simulink model "ackerman_modelo_parte1_neuronal"  (R2023b)
settings: Solver=FixedStepDiscrete  StartTime=0.0  StopTime=50  FixedStep=0.1  RelTol=1e-3
undefined symbols (not defined in the file or in its folder): Angular, Linear
libraries: neural x121, robotlib x15, fuzblock x1, robotcorelib x1
(part 5 of 5)

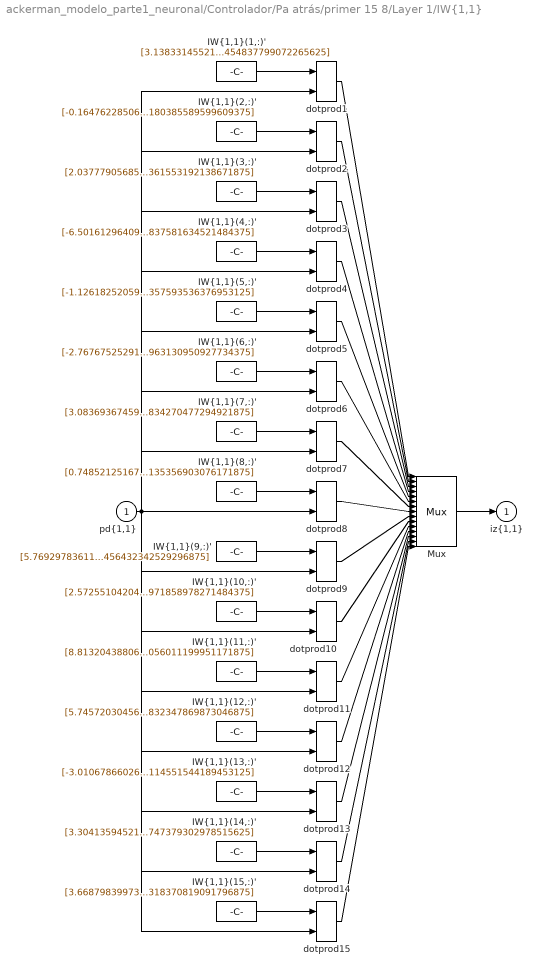
== system ackerman_modelo_parte1_neuronal/Controlador/Pa atrás/primer 15 8/Layer 1/IW{1,1} ==
  "pd{1,1}" : Inport  PortDimensions=12  SampleTime=0.1
      mask Display: e = 0.06;c1 = [120 230 180]/255;c2 = ([120 230 180]+0)/(256+128);c3 = ([120 230 180]+128)/(256+128);patch([0 1 1 0],[0 0 1 1],c1);patch([0 1 1 1-e 1-e 0+e],[0 0 1 1-e 0+e 0+e],c2);patch([0 0 1 1-e 0+e 0+e],[0 1 1 1-e 1-e 0+e],c3);plot([0 1 1 0 0],[0 0 1 1 0]);
  "IW{1,1}(1,:)'" : Constant  Value=[3.13833145521684198087086770101450383663177490234375;-6.19499437988781220809642036329023540019989013671875;-2.00220395313596899455887978547252714633941650390625;-4.82784976961187251021101474179886281490325927734375;5.58430706351398686848597208154387772083282470703125;5.3963459231659864911989643587730824947357177734375;0.0542977229144951945016828176449052989482879638671875;-4.8964896730979479144707511295564472675323486328125;1.547154767949700637785781509592197835445404052734375;7.9004335446761420058692237944342195987701416015625;4.14971538332680278671205087448470294475555419921875;-0.79014433640509429412901454270468093454837799072265625]
      mask Display: e = 0.06;c1 = [120 150 230]/255;c2 = ([120 150 230]+0)/383;c3 = ([120 150 230]+128)/383;patch([0 1 1 0],[0 0 1 1],c1);patch([0 1 1 1-e 1-e 0+e],[0 0 1 1-e 0+e 0+e],c2);patch([0 0 1 1-e 0+e 0+e],[0 1 1 1-e 1-e 0+e],c3);plot([0 1 1 0 0],[0 0 1 1 0]);disp('Weights');
  "IW{1,1}(10,:)'" : Constant  Value=[2.572551042042926727759777350001968443393707275390625;-0.59551225184145584190531508284038864076137542724609375;-0.30685873733525692585999422590248286724090576171875;-2.6996858864094601671013151644729077816009521484375;-4.249827912405418572916460107080638408660888671875;-1.1549695122995402574161971642752178013324737548828125;-13.3261726054552465114966253167949616909027099609375;4.43615378343977084796279086731374263763427734375;0.5770168591797031343304524853010661900043487548828125;0.27150941942864859068862415369949303567409515380859375;3.406433890218272697580914609716273844242095947265625;0.92716581704404477104475290616392157971858978271484375]
      mask Display: e = 0.06;c1 = [120 150 230]/255;c2 = ([120 150 230]+0)/383;c3 = ([120 150 230]+128)/383;patch([0 1 1 0],[0 0 1 1],c1);patch([0 1 1 1-e 1-e 0+e],[0 0 1 1-e 0+e 0+e],c2);patch([0 0 1 1-e 0+e 0+e],[0 1 1 1-e 1-e 0+e],c3);plot([0 1 1 0 0],[0 0 1 1 0]);disp('Weights');
  "IW{1,1}(11,:)'" : Constant  Value=[8.813204388067607197854158584959805011749267578125;-11.7057265338999574311174001195468008518218994140625;-1.1611569417966640660466737244860269129276275634765625;-0.282140073577483274647192956763319671154022216796875;-6.070085924028401080931871547363698482513427734375;-1.1869447949154434684970738089759834110736846923828125;12.797002497650527885753035661764442920684814453125;-6.5006412352421936162727433838881552219390869140625;2.544454447903282900966814850107766687870025634765625;2.772478853294586986777403581072576344013214111328125;3.09454714741394543153774066013284027576446533203125;7.86219239038993134016664043883793056011199951171875]
      mask Display: e = 0.06;c1 = [120 150 230]/255;c2 = ([120 150 230]+0)/383;c3 = ([120 150 230]+128)/383;patch([0 1 1 0],[0 0 1 1],c1);patch([0 1 1 1-e 1-e 0+e],[0 0 1 1-e 0+e 0+e],c2);patch([0 0 1 1-e 0+e 0+e],[0 1 1 1-e 1-e 0+e],c3);plot([0 1 1 0 0],[0 0 1 1 0]);disp('Weights');
  "IW{1,1}(12,:)'" : Constant  Value=[5.7457203045610523162167737609706819057464599609375;-4.95127673804246715150156887830235064029693603515625;-2.57218520303488151768078751047141849994659423828125;-0.73249175551907896863923497221549041569232940673828125;1.6111606945435188453785713136312551796436309814453125;1.1705981175054331888674141737283207476139068603515625;-7.34947786476711684144902392290532588958740234375;-1.7738172654386639148782478514476679265499114990234375;0.5768042451301245154837715745088644325733184814453125;0.224641956192956959714734921362833119928836822509765625;0.3930249748530252329459244720055721700191497802734375;-1.5133229059635364688318759363028220832347869873046875]
      mask Display: e = 0.06;c1 = [120 150 230]/255;c2 = ([120 150 230]+0)/383;c3 = ([120 150 230]+128)/383;patch([0 1 1 0],[0 0 1 1],c1);patch([0 1 1 1-e 1-e 0+e],[0 0 1 1-e 0+e 0+e],c2);patch([0 0 1 1-e 0+e 0+e],[0 1 1 1-e 1-e 0+e],c3);plot([0 1 1 0 0],[0 0 1 1 0]);disp('Weights');
  "IW{1,1}(13,:)'" : Constant  Value=[-3.010678660268370609998100917437113821506500244140625;4.4328891620700812126187884132377803325653076171875;5.807431661847648030061463941819965839385986328125;3.476791359428748950932686057058162987232208251953125;2.4697341429991155337120289914309978485107421875;2.05477310015384961872086932999081909656524658203125;-1.5218585447957073686353623998002149164676666259765625;1.324210651061530352734507687273435294628143310546875;5.75386815156350195366030675359070301055908203125;5.10401477499944977722634575911797583103179931640625;1.7878470401743256079640786992968060076236724853515625;-1.4389725445316703389408985458430834114551544189453125]
      mask Display: e = 0.06;c1 = [120 150 230]/255;c2 = ([120 150 230]+0)/383;c3 = ([120 150 230]+128)/383;patch([0 1 1 0],[0 0 1 1],c1);patch([0 1 1 1-e 1-e 0+e],[0 0 1 1-e 0+e 0+e],c2);patch([0 0 1 1-e 0+e 0+e],[0 1 1 1-e 1-e 0+e],c3);plot([0 1 1 0 0],[0 0 1 1 0]);disp('Weights');
  "IW{1,1}(14,:)'" : Constant  Value=[3.3041359452168297394791807164438068866729736328125;0.1762778979927372702274368521102587692439556121826171875;5.4050963927401287634211257682181894779205322265625;-3.18648301109764275906854891218245029449462890625;0.5385228763760065984200764432898722589015960693359375;-2.302199268748124527661502725095488131046295166015625;5.49227092147563933366427590954117476940155029296875;0.97919070401553154336937723201117478311061859130859375;1.145084516988541967208448113524354994297027587890625;4.27032650445300010488836051081307232379913330078125;1.6231956725708138744579400736256502568721771240234375;-0.6865005967335078285174176926375366747379302978515625]
      mask Display: e = 0.06;c1 = [120 150 230]/255;c2 = ([120 150 230]+0)/383;c3 = ([120 150 230]+128)/383;patch([0 1 1 0],[0 0 1 1],c1);patch([0 1 1 1-e 1-e 0+e],[0 0 1 1-e 0+e 0+e],c2);patch([0 0 1 1-e 0+e 0+e],[0 1 1 1-e 1-e 0+e],c3);plot([0 1 1 0 0],[0 0 1 1 0]);disp('Weights');
  "IW{1,1}(15,:)'" : Constant  Value=[3.668798399734122472892750010942108929157257080078125;-5.38938465059415960922706290148198604583740234375;-3.401566331543757204514122349792160093784332275390625;-1.1609126490613366211590573584544472396373748779296875;6.618010649271667489301762543618679046630859375;-7.862741094876252390122317592613399028778076171875;3.54191550708989755236189012066461145877838134765625;-1.3477909930119469361642359217512421309947967529296875;1.9546134173191365146493581050890497863292694091796875;-1.1566749706934935648661166851525194942951202392578125;2.921489032247831740818355683586560189723968505859375;1.5151945125394365998516832405584864318370819091796875]
      mask Display: e = 0.06;c1 = [120 150 230]/255;c2 = ([120 150 230]+0)/383;c3 = ([120 150 230]+128)/383;patch([0 1 1 0],[0 0 1 1],c1);patch([0 1 1 1-e 1-e 0+e],[0 0 1 1-e 0+e 0+e],c2);patch([0 0 1 1-e 0+e 0+e],[0 1 1 1-e 1-e 0+e],c3);plot([0 1 1 0 0],[0 0 1 1 0]);disp('Weights');
  "IW{1,1}(2,:)'" : Constant  Value=[-0.1647622850618779555276205428526736795902252197265625;-6.67270935708041523781730575137771666049957275390625;-1.6748440892445206618077691018697805702686309814453125;0.97276097993890042747722191052162088453769683837890625;2.73413105911384235469085979275405406951904296875;-4.61712661552317182867000155965797603130340576171875;-2.911426019223313677031228507985360920429229736328125;0.72363976938584340103943759459070861339569091796875;-0.98313354310142819780793388417805545032024383544921875;-2.691014741691610812068802260910160839557647705078125;4.420274579392863500970634049735963344573974609375;-3.880848224433525839316416750079952180385589599609375]
      mask Display: e = 0.06;c1 = [120 150 230]/255;c2 = ([120 150 230]+0)/383;c3 = ([120 150 230]+128)/383;patch([0 1 1 0],[0 0 1 1],c1);patch([0 1 1 1-e 1-e 0+e],[0 0 1 1-e 0+e 0+e],c2);patch([0 0 1 1-e 0+e 0+e],[0 1 1 1-e 1-e 0+e],c3);plot([0 1 1 0 0],[0 0 1 1 0]);disp('Weights');
  "IW{1,1}(3,:)'" : Constant  Value=[2.03777905685296989446442239568568766117095947265625;-2.160035947260035005257350348983891308307647705078125;2.605648632233163564109190701856277883052825927734375;2.3092568544783862449776279390789568424224853515625;3.3144277547602793987380209728144109249114990234375;-2.28108752553862448309018873260356485843658447265625;-10.7986674070768398081554551026783883571624755859375;3.853720755030112687933296911069191992282867431640625;-2.361428195660809858935635929810814559459686279296875;-3.596462160164643595550160171114839613437652587890625;-3.910945166775002146408724001958034932613372802734375;-2.429732741520268302082286027143709361553192138671875]
      mask Display: e = 0.06;c1 = [120 150 230]/255;c2 = ([120 150 230]+0)/383;c3 = ([120 150 230]+128)/383;patch([0 1 1 0],[0 0 1 1],c1);patch([0 1 1 1-e 1-e 0+e],[0 0 1 1-e 0+e 0+e],c2);patch([0 0 1 1-e 0+e 0+e],[0 1 1 1-e 1-e 0+e],c3);plot([0 1 1 0 0],[0 0 1 1 0]);disp('Weights');
  "IW{1,1}(4,:)'" : Constant  Value=[-6.5016129640967559311093282303772866725921630859375;-0.79522721813868890716747728220070712268352508544921875;-6.73803458296746260458576216478832066059112548828125;-3.476541997292326602320144957047887146472930908203125;-2.55914140829384084696584977791644632816314697265625;-3.88475771154622950831480920896865427494049072265625;-1.4635945598190376326641626292257569730281829833984375;3.299453679629163360687016393058001995086669921875;3.0582672371355261731196151231415569782257080078125;-0.57414285366964612489226738034631125628948211669921875;0.93060935916938891665495248162187635898590087890625;-0.429906101754307046203251729821204207837581634521484375]
      mask Display: e = 0.06;c1 = [120 150 230]/255;c2 = ([120 150 230]+0)/383;c3 = ([120 150 230]+128)/383;patch([0 1 1 0],[0 0 1 1],c1);patch([0 1 1 1-e 1-e 0+e],[0 0 1 1-e 0+e 0+e],c2);patch([0 0 1 1-e 0+e 0+e],[0 1 1 1-e 1-e 0+e],c3);plot([0 1 1 0 0],[0 0 1 1 0]);disp('Weights');
  "IW{1,1}(5,:)'" : Constant  Value=[-1.126182520599181113851727786823175847530364990234375;-0.67009231564694093918888029293157160282135009765625;2.990487179943574158613728286582045257091522216796875;1.686459004262194749657055581337772309780120849609375;-0.51295798280588311701677639575791545212268829345703125;-0.1693192751783541283305822844340582378208637237548828125;-3.36835087006842837098474774393253028392791748046875;3.730050960124993597588627380901016294956207275390625;1.9196643529733361521749657185864634811878204345703125;1.694496082969093375680813551298342645168304443359375;-1.0729297441333509599559192793094553053379058837890625;-2.796374710798151586033100102213211357593536376953125]
      mask Display: e = 0.06;c1 = [120 150 230]/255;c2 = ([120 150 230]+0)/383;c3 = ([120 150 230]+128)/383;patch([0 1 1 0],[0 0 1 1],c1);patch([0 1 1 1-e 1-e 0+e],[0 0 1 1-e 0+e 0+e],c2);patch([0 0 1 1-e 0+e 0+e],[0 1 1 1-e 1-e 0+e],c3);plot([0 1 1 0 0],[0 0 1 1 0]);disp('Weights');
  "IW{1,1}(6,:)'" : Constant  Value=[-2.767675252918380568445400058408267796039581298828125;-7.073354838042828163224839954636991024017333984375;-1.3531578339525538456911135654081590473651885986328125;-3.06300573535806019975780145614407956600189208984375;-7.13075550648704403755573366652242839336395263671875;-3.744633843247024973521774882101453840732574462890625;-8.208592620912252613152304547838866710662841796875;2.46583543118132553217947133816778659820556640625;-3.340073357912283658066598945879377424716949462890625;-2.799475440893957500776423330535180866718292236328125;-2.249013441580913319484125167946331202983856201171875;2.392302749944286599514953195466659963130950927734375]
      mask Display: e = 0.06;c1 = [120 150 230]/255;c2 = ([120 150 230]+0)/383;c3 = ([120 150 230]+128)/383;patch([0 1 1 0],[0 0 1 1],c1);patch([0 1 1 1-e 1-e 0+e],[0 0 1 1-e 0+e 0+e],c2);patch([0 0 1 1-e 0+e 0+e],[0 1 1 1-e 1-e 0+e],c3);plot([0 1 1 0 0],[0 0 1 1 0]);disp('Weights');
  "IW{1,1}(7,:)'" : Constant  Value=[3.0836936745987717500838698470033705234527587890625;-0.88318704317611373966201426810584962368011474609375;1.7110761895791217757079039074596948921680450439453125;-0.31400445778907759564191337631200440227985382080078125;2.64346625227536247138004910084418952465057373046875;-0.6176657494047643748302789390436373651027679443359375;-0.63152317856311934729518497988465242087841033935546875;8.3510900927338820309842049027793109416961669921875;-5.97435811941152916659802940557710826396942138671875;-0.6339005945491880122943939568358473479747772216796875;2.279868767326854506194422356202267110347747802734375;-3.37930106039398037154342091525904834270477294921875]
      mask Display: e = 0.06;c1 = [120 150 230]/255;c2 = ([120 150 230]+0)/383;c3 = ([120 150 230]+128)/383;patch([0 1 1 0],[0 0 1 1],c1);patch([0 1 1 1-e 1-e 0+e],[0 0 1 1-e 0+e 0+e],c2);patch([0 0 1 1-e 0+e 0+e],[0 1 1 1-e 1-e 0+e],c3);plot([0 1 1 0 0],[0 0 1 1 0]);disp('Weights');
  "IW{1,1}(8,:)'" : Constant  Value=[0.74852125167156613461116876351297833025455474853515625;-4.012567271762879528296252829022705554962158203125;1.0633341155585138704253722607973031699657440185546875;-0.58494336521590450939100946925464086234569549560546875;-0.5453224736011679230074378210701979696750640869140625;3.469959956693179581321828663931228220462799072265625;-5.89367912672649563177174059092067182064056396484375;-4.74017192421732413976087627816013991832733154296875;-4.9750537290780183496963218203745782375335693359375;6.49748859653846633221974116167984902858734130859375;-1.910694940986072065669532094034366309642791748046875;-2.236924241129784274306757652084343135356903076171875]
      mask Display: e = 0.06;c1 = [120 150 230]/255;c2 = ([120 150 230]+0)/383;c3 = ([120 150 230]+128)/383;patch([0 1 1 0],[0 0 1 1],c1);patch([0 1 1 1-e 1-e 0+e],[0 0 1 1-e 0+e 0+e],c2);patch([0 0 1 1-e 0+e 0+e],[0 1 1 1-e 1-e 0+e],c3);plot([0 1 1 0 0],[0 0 1 1 0]);disp('Weights');
  "IW{1,1}(9,:)'" : Constant  Value=[5.76929783611728819181507788016460835933685302734375;0.85907947622363323159078163371304981410503387451171875;-1.0414871446960243250856592567288316786289215087890625;-0.60378548209747384678536263891146518290042877197265625;1.936814065109272231524073504260741174221038818359375;5.14869148164522183463986948481760919094085693359375;-1.94708708587885492846680790535174310207366943359375;-0.52074196027196240077472566554206423461437225341796875;1.6221727344143810345400424921535886824131011962890625;-1.153231367094303738696225991589017212390899658203125;0.47589760448268070280875008393195457756519317626953125;1.595810956015813797392866035806946456432342529296875]
      mask Display: e = 0.06;c1 = [120 150 230]/255;c2 = ([120 150 230]+0)/383;c3 = ([120 150 230]+128)/383;patch([0 1 1 0],[0 0 1 1],c1);patch([0 1 1 1-e 1-e 0+e],[0 0 1 1-e 0+e 0+e],c2);patch([0 0 1 1-e 0+e 0+e],[0 1 1 1-e 1-e 0+e],c3);plot([0 1 1 0 0],[0 0 1 1 0]);disp('Weights');
  Mux : Mux  Inputs=15
      mask Display: e = 0.06;c1 = [120 150 230]/255;c2 = ([120 150 230]+0)/383;c3 = ([120 150 230]+128)/383;patch([0 1 1 0],[0 0 1 1],c1);patch([0 1 1 1-e 1-e 0+e],[0 0 1 1-e 0+e 0+e],c2);patch([0 0 1 1-e 0+e 0+e],[0 1 1 1-e 1-e 0+e],c3);plot([0 1 1 0 0],[0 0 1 1 0]);disp('Mux');
  dotprod{1..15} (15 alike) : neural/Weight Functions/dotprod
  "iz{1,1}" : Outport
      mask Display: e = 0.06;c1 = [120 230 180]/255;c2 = ([120 230 180]+0)/(256+128);c3 = ([120 230 180]+128)/(256+128);patch([0 1 1 0],[0 0 1 1],c1);patch([0 1 1 1-e 1-e 0+e],[0 0 1 1-e 0+e 0+e],c2);patch([0 0 1 1-e 0+e 0+e],[0 1 1 1-e 1-e 0+e],c3);plot([0 1 1 0 0],[0 0 1 1 0]);
  wires:
  Mux/1 -> "iz{1,1}"/1
  dotprod15/1 -> Mux/15
  "IW{1,1}(15,:)'"/1 -> dotprod15/1
  dotprod14/1 -> Mux/14
  "IW{1,1}(14,:)'"/1 -> dotprod14/1
  dotprod13/1 -> Mux/13
  "IW{1,1}(13,:)'"/1 -> dotprod13/1
  dotprod12/1 -> Mux/12
  "IW{1,1}(12,:)'"/1 -> dotprod12/1
  dotprod11/1 -> Mux/11
  "IW{1,1}(11,:)'"/1 -> dotprod11/1
  dotprod10/1 -> Mux/10
  "IW{1,1}(10,:)'"/1 -> dotprod10/1
  dotprod9/1 -> Mux/9
  "IW{1,1}(9,:)'"/1 -> dotprod9/1
  dotprod8/1 -> Mux/8
  "IW{1,1}(8,:)'"/1 -> dotprod8/1
  dotprod7/1 -> Mux/7
  "IW{1,1}(7,:)'"/1 -> dotprod7/1
  dotprod6/1 -> Mux/6
  "IW{1,1}(6,:)'"/1 -> dotprod6/1
  dotprod5/1 -> Mux/5
  "IW{1,1}(5,:)'"/1 -> dotprod5/1
  dotprod4/1 -> Mux/4
  "IW{1,1}(4,:)'"/1 -> dotprod4/1
  dotprod3/1 -> Mux/3
  "IW{1,1}(3,:)'"/1 -> dotprod3/1
  dotprod2/1 -> Mux/2
  "IW{1,1}(2,:)'"/1 -> dotprod2/1
  dotprod1/1 -> Mux/1
  "pd{1,1}"/1 -> dotprod15/2, dotprod14/2, dotprod13/2, dotprod12/2, dotprod11/2, dotprod10/2, dotprod9/2, dotprod8/2, dotprod7/2, dotprod6/2, dotprod5/2, dotprod4/2, dotprod3/2, dotprod2/2, dotprod1/2
  "IW{1,1}(1,:)'"/1 -> dotprod1/1

== system ackerman_modelo_parte1_neuronal/Controlador/Pa atrás/primer 15 8/Layer 2/Delays 1 ==
  "p{2}" : Inport  PortDimensions=15  SampleTime=0.1
      mask Display: e = 0.06;c1 = [120 230 180]/255;c2 = ([120 230 180]+0)/(256+128);c3 = ([120 230 180]+128)/(256+128);patch([0 1 1 0],[0 0 1 1],c1);patch([0 1 1 1-e 1-e 0+e],[0 0 1 1-e 0+e 0+e],c2);patch([0 0 1 1-e 0+e 0+e],[0 1 1 1-e 1-e 0+e],c3);plot([0 1 1 0 0],[0 0 1 1 0]);
  mux : Mux  Inputs=1
      mask Display: e = 0.06;c1 = [120 150 230]/255;c2 = ([120 150 230]+0)/383;c3 = ([120 150 230]+128)/383;patch([0 1 1 0],[0 0 1 1],c1);patch([0 1 1 1-e 1-e 0+e],[0 0 1 1-e 0+e 0+e],c2);patch([0 0 1 1-e 0+e 0+e],[0 1 1 1-e 1-e 0+e],c3);plot([0 1 1 0 0],[0 0 1 1 0]);disp('Mux')
  "pd{2,1}" : Outport
      mask Display: e = 0.06;c1 = [120 230 180]/255;c2 = ([120 230 180]+0)/(256+128);c3 = ([120 230 180]+128)/(256+128);patch([0 1 1 0],[0 0 1 1],c1);patch([0 1 1 1-e 1-e 0+e],[0 0 1 1-e 0+e 0+e],c2);patch([0 0 1 1-e 0+e 0+e],[0 1 1 1-e 1-e 0+e],c3);plot([0 1 1 0 0],[0 0 1 1 0]);
  wires:
  mux/1 -> "pd{2,1}"/1
  "p{2}"/1 -> mux/1

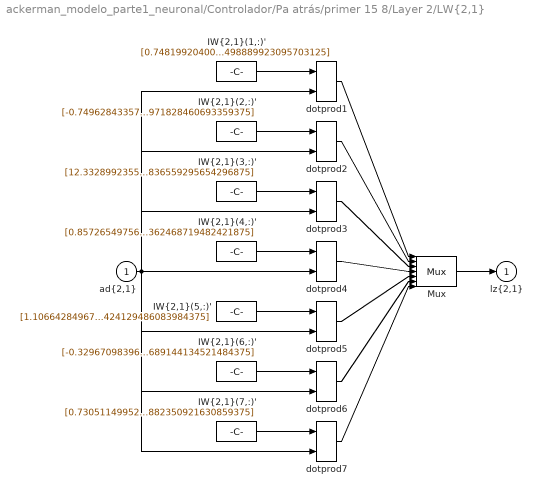
== system ackerman_modelo_parte1_neuronal/Controlador/Pa atrás/primer 15 8/Layer 2/LW{2,1} ==
  "ad{2,1}" : Inport  PortDimensions=15  SampleTime=0.1
      mask Display: e = 0.06;c1 = [120 230 180]/255;c2 = ([120 230 180]+0)/(256+128);c3 = ([120 230 180]+128)/(256+128);patch([0 1 1 0],[0 0 1 1],c1);patch([0 1 1 1-e 1-e 0+e],[0 0 1 1-e 0+e 0+e],c2);patch([0 0 1 1-e 0+e 0+e],[0 1 1 1-e 1-e 0+e],c3);plot([0 1 1 0 0],[0 0 1 1 0]);
  "IW{2,1}(1,:)'" : Constant  Value=[0.7481992040039153746278088874532841145992279052734375;-1.126597024044754480343044633627869188785552978515625;1.5155775237853175152480389442644082009792327880859375;2.0469156099994307851375197060406208038330078125;7.8138659751533072750362407532520592212677001953125;2.903583859678425138639568103826604783535003662109375;1.6622982814302422749364041010267101228237152099609375;5.9303213640288259256294622900895774364471435546875;-4.31311558360107927256876791943795979022979736328125;-8.8773576403826783831618740805424749851226806640625;-4.04397070113652556955230465973727405071258544921875;-5.08185092549631800551424021250568330287933349609375;-2.80925265953370395521915270364843308925628662109375;-1.864831680495824262067117160768248140811920166015625;2.65513075966677281058991866302676498889923095703125]
      mask Display: e = 0.06;c1 = [120 150 230]/255;c2 = ([120 150 230]+0)/383;c3 = ([120 150 230]+128)/383;patch([0 1 1 0],[0 0 1 1],c1);patch([0 1 1 1-e 1-e 0+e],[0 0 1 1-e 0+e 0+e],c2);patch([0 0 1 1-e 0+e 0+e],[0 1 1 1-e 1-e 0+e],c3);plot([0 1 1 0 0],[0 0 1 1 0]);disp('weights');
  "IW{2,1}(2,:)'" : Constant  Value=[-0.74962843357484931772205527522601187229156494140625;-6.93165936727352960389225700055249035358428955078125;-4.01275508893955379363660540548153221607208251953125;-2.120531649750461600234530123998410999774932861328125;1.829294262234303136693824853864498436450958251953125;6.57831915986466153611900153919123113155364990234375;3.111129228600808982463377105887047946453094482421875;-1.906397126721314894126635408611036837100982666015625;-2.561940433343730116888536940678022801876068115234375;3.701734633273577212975169459241442382335662841796875;2.456765678314351664113246442866511642932891845703125;-0.88958234176935591097645783520420081913471221923828125;-6.4768830231558265353442038758657872676849365234375;4.57889656160470082113533862866461277008056640625;4.0829006341815610170442596427164971828460693359375]
      mask Display: e = 0.06;c1 = [120 150 230]/255;c2 = ([120 150 230]+0)/383;c3 = ([120 150 230]+128)/383;patch([0 1 1 0],[0 0 1 1],c1);patch([0 1 1 1-e 1-e 0+e],[0 0 1 1-e 0+e 0+e],c2);patch([0 0 1 1-e 0+e 0+e],[0 1 1 1-e 1-e 0+e],c3);plot([0 1 1 0 0],[0 0 1 1 0]);disp('weights');
  "IW{2,1}(3,:)'" : Constant  Value=[12.3328992355445858919438251177780330181121826171875;11.0004326759787804945744937867857515811920166015625;-5.34841924221345532686200385796837508678436279296875;-7.0994335148749936337253529927693307399749755859375;2.263077368879132134082965421839617192745208740234375;-7.31242298972578996796300998539663851261138916015625;9.365048931524153630334694753400981426239013671875;3.968973565914051704339726711623370647430419921875;15.059144497544654228704530396498739719390869140625;6.4716573827061711909891528193838894367218017578125;-5.9158271638871067210629917099140584468841552734375;-3.05024650789953444274260618840344250202178955078125;8.2370518811566935113432919024489820003509521484375;-11.6324162769302521525105476030148565769195556640625;2.01322611861408784506011215853504836559295654296875]
      mask Display: e = 0.06;c1 = [120 150 230]/255;c2 = ([120 150 230]+0)/383;c3 = ([120 150 230]+128)/383;patch([0 1 1 0],[0 0 1 1],c1);patch([0 1 1 1-e 1-e 0+e],[0 0 1 1-e 0+e 0+e],c2);patch([0 0 1 1-e 0+e 0+e],[0 1 1 1-e 1-e 0+e],c3);plot([0 1 1 0 0],[0 0 1 1 0]);disp('weights');
  "IW{2,1}(4,:)'" : Constant  Value=[0.85726549756485825870555572691955603659152984619140625;-1.6157874357042329993561224910081364214420318603515625;-2.3378881600398013773656202829442918300628662109375;1.4068312031528831251847577732405625283718109130859375;1.1609880290264327218352491399855352938175201416015625;5.043137081505467023134769988246262073516845703125;1.6282908256337644825606503218295983970165252685546875;0.9851818610864018221917604023474268615245819091796875;-1.5742354980467549996347997876000590622425079345703125;-6.4182878725017058485491361352615058422088623046875;1.236131349069788054606533478363417088985443115234375;-1.5151875690311220612471743152127601206302642822265625;-5.4046776681074533144055749289691448211669921875;-0.301835111587298310364957387719186954200267791748046875;-1.662398546290766443433994936640374362468719482421875]
      mask Display: e = 0.06;c1 = [120 150 230]/255;c2 = ([120 150 230]+0)/383;c3 = ([120 150 230]+128)/383;patch([0 1 1 0],[0 0 1 1],c1);patch([0 1 1 1-e 1-e 0+e],[0 0 1 1-e 0+e 0+e],c2);patch([0 0 1 1-e 0+e 0+e],[0 1 1 1-e 1-e 0+e],c3);plot([0 1 1 0 0],[0 0 1 1 0]);disp('weights');
  "IW{2,1}(5,:)'" : Constant  Value=[1.106642849674602135934264879324473440647125244140625;0.571502015897777937425416894257068634033203125;0.81620295508666396155916800125851295888423919677734375;-3.915085877175725759258284597308374941349029541015625;1.7182548217798458978222697624005377292633056640625;-0.932288532598022801067827458609826862812042236328125;-3.802149167051169786901709812809713184833526611328125;1.1218625349822100023544635405414737761020660400390625;1.2108603063697682689081602802616544067859649658203125;-1.3837647454165533655867648121784441173076629638671875;-2.294782958455342747328131736139766871929168701171875;0.27139709347339202594184826011769473552703857421875;0.35111556880865635310584593753446824848651885986328125;-0.535119520474186316505438298918306827545166015625;0.177795112653033215988074289271025918424129486083984375]
      mask Display: e = 0.06;c1 = [120 150 230]/255;c2 = ([120 150 230]+0)/383;c3 = ([120 150 230]+128)/383;patch([0 1 1 0],[0 0 1 1],c1);patch([0 1 1 1-e 1-e 0+e],[0 0 1 1-e 0+e 0+e],c2);patch([0 0 1 1-e 0+e 0+e],[0 1 1 1-e 1-e 0+e],c3);plot([0 1 1 0 0],[0 0 1 1 0]);disp('weights');
  "IW{2,1}(6,:)'" : Constant  Value=[-0.329670983964105934749255766291753388941287994384765625;0.9447396245833641348355058653396554291248321533203125;-0.260196034449015456413434321802924387156963348388671875;-0.2872857726077722162472127820365130901336669921875;2.91913437532715480671186014660634100437164306640625;0.1852331668108104789638446163735352456569671630859375;0.68985458226234264156317976812715642154216766357421875;-1.7856832233152906130868586842552758753299713134765625;-0.44000187852971850421823774013319052755832672119140625;-2.142873037757759835386650593136437237262725830078125;0.388272349961649665406326903394074179232120513916015625;-0.60718998768551724065645203154417686164379119873046875;0.8371629651469361110827094307751394808292388916015625;0.1650951326068933744384281681050197221338748931884765625;0.64000300449640989963739912127493880689144134521484375]
      mask Display: e = 0.06;c1 = [120 150 230]/255;c2 = ([120 150 230]+0)/383;c3 = ([120 150 230]+128)/383;patch([0 1 1 0],[0 0 1 1],c1);patch([0 1 1 1-e 1-e 0+e],[0 0 1 1-e 0+e 0+e],c2);patch([0 0 1 1-e 0+e 0+e],[0 1 1 1-e 1-e 0+e],c3);plot([0 1 1 0 0],[0 0 1 1 0]);disp('weights');
  "IW{2,1}(7,:)'" : Constant  Value=[0.73051149952431082557069430549745447933673858642578125;3.05826356477004512868234087363816797733306884765625;-1.673669437076252819451838149689137935638427734375;-2.400459004009674490731640617013908922672271728515625;-9.80319466489697077804521541111171245574951171875;4.62435712954842959021561910049058496952056884765625;-4.84177000897603448947847937233746051788330078125;-8.425474797648991653886696440167725086212158203125;-3.37578421790337568353379538166336715221405029296875;-3.11041385548329518684340655454434454441070556640625;2.677786696924715936773964131134562194347381591796875;3.9061912060113375133596491650678217411041259765625;1.013606829036505008190260923583991825580596923828125;4.45431275129676151891544577665627002716064453125;-10.9998218846045059393645715317688882350921630859375]
      mask Display: e = 0.06;c1 = [120 150 230]/255;c2 = ([120 150 230]+0)/383;c3 = ([120 150 230]+128)/383;patch([0 1 1 0],[0 0 1 1],c1);patch([0 1 1 1-e 1-e 0+e],[0 0 1 1-e 0+e 0+e],c2);patch([0 0 1 1-e 0+e 0+e],[0 1 1 1-e 1-e 0+e],c3);plot([0 1 1 0 0],[0 0 1 1 0]);disp('weights');
  Mux : Mux  Inputs=7
      mask Display: e = 0.06;c1 = [120 150 230]/255;c2 = ([120 150 230]+0)/383;c3 = ([120 150 230]+128)/383;patch([0 1 1 0],[0 0 1 1],c1);patch([0 1 1 1-e 1-e 0+e],[0 0 1 1-e 0+e 0+e],c2);patch([0 0 1 1-e 0+e 0+e],[0 1 1 1-e 1-e 0+e],c3);plot([0 1 1 0 0],[0 0 1 1 0]);disp('Mux');
  dotprod{1..7} (7 alike) : neural/Weight Functions/dotprod
  "lz{2,1}" : Outport
      mask Display: e = 0.06;c1 = [120 230 180]/255;c2 = ([120 230 180]+0)/(256+128);c3 = ([120 230 180]+128)/(256+128);patch([0 1 1 0],[0 0 1 1],c1);patch([0 1 1 1-e 1-e 0+e],[0 0 1 1-e 0+e 0+e],c2);patch([0 0 1 1-e 0+e 0+e],[0 1 1 1-e 1-e 0+e],c3);plot([0 1 1 0 0],[0 0 1 1 0]);
  wires:
  Mux/1 -> "lz{2,1}"/1
  dotprod7/1 -> Mux/7
  "IW{2,1}(7,:)'"/1 -> dotprod7/1
  dotprod6/1 -> Mux/6
  "IW{2,1}(6,:)'"/1 -> dotprod6/1
  dotprod5/1 -> Mux/5
  "IW{2,1}(5,:)'"/1 -> dotprod5/1
  dotprod4/1 -> Mux/4
  "IW{2,1}(4,:)'"/1 -> dotprod4/1
  dotprod3/1 -> Mux/3
  "IW{2,1}(3,:)'"/1 -> dotprod3/1
  dotprod2/1 -> Mux/2
  "IW{2,1}(2,:)'"/1 -> dotprod2/1
  dotprod1/1 -> Mux/1
  "ad{2,1}"/1 -> dotprod7/2, dotprod6/2, dotprod5/2, dotprod4/2, dotprod3/2, dotprod2/2, dotprod1/2
  "IW{2,1}(1,:)'"/1 -> dotprod1/1

== system ackerman_modelo_parte1_neuronal/Controlador/Pa atrás/primer 15 8/Layer 3/Delays 1 ==
  "p{3}" : Inport  PortDimensions=7  SampleTime=0.1
      mask Display: e = 0.06;c1 = [120 230 180]/255;c2 = ([120 230 180]+0)/(256+128);c3 = ([120 230 180]+128)/(256+128);patch([0 1 1 0],[0 0 1 1],c1);patch([0 1 1 1-e 1-e 0+e],[0 0 1 1-e 0+e 0+e],c2);patch([0 0 1 1-e 0+e 0+e],[0 1 1 1-e 1-e 0+e],c3);plot([0 1 1 0 0],[0 0 1 1 0]);
  mux : Mux  Inputs=1
      mask Display: e = 0.06;c1 = [120 150 230]/255;c2 = ([120 150 230]+0)/383;c3 = ([120 150 230]+128)/383;patch([0 1 1 0],[0 0 1 1],c1);patch([0 1 1 1-e 1-e 0+e],[0 0 1 1-e 0+e 0+e],c2);patch([0 0 1 1-e 0+e 0+e],[0 1 1 1-e 1-e 0+e],c3);plot([0 1 1 0 0],[0 0 1 1 0]);disp('Mux')
  "pd{3,2}" : Outport
      mask Display: e = 0.06;c1 = [120 230 180]/255;c2 = ([120 230 180]+0)/(256+128);c3 = ([120 230 180]+128)/(256+128);patch([0 1 1 0],[0 0 1 1],c1);patch([0 1 1 1-e 1-e 0+e],[0 0 1 1-e 0+e 0+e],c2);patch([0 0 1 1-e 0+e 0+e],[0 1 1 1-e 1-e 0+e],c3);plot([0 1 1 0 0],[0 0 1 1 0]);
  wires:
  mux/1 -> "pd{3,2}"/1
  "p{3}"/1 -> mux/1

== system ackerman_modelo_parte1_neuronal/Controlador/Pa atrás/primer 15 8/Layer 3/LW{3,2} ==
  "ad{3,2}" : Inport  PortDimensions=7  SampleTime=0.1
      mask Display: e = 0.06;c1 = [120 230 180]/255;c2 = ([120 230 180]+0)/(256+128);c3 = ([120 230 180]+128)/(256+128);patch([0 1 1 0],[0 0 1 1],c1);patch([0 1 1 1-e 1-e 0+e],[0 0 1 1-e 0+e 0+e],c2);patch([0 0 1 1-e 0+e 0+e],[0 1 1 1-e 1-e 0+e],c3);plot([0 1 1 0 0],[0 0 1 1 0]);
  "IW{3,2}(1,:)'" : Constant  Value=[-0.264079440465544046379164910831605084240436553955078125;0.51230046191857103732303357901400886476039886474609375;-0.6652775182707999501730000702082179486751556396484375;-0.53484339021644611289474369186791591346263885498046875;-0.149228947666670774818697964292368851602077484130859375;-0.008433135735000978072672950247579137794673442840576171875;-0.85256293215924350281653687488869763910770416259765625]
      mask Display: e = 0.06;c1 = [120 150 230]/255;c2 = ([120 150 230]+0)/383;c3 = ([120 150 230]+128)/383;patch([0 1 1 0],[0 0 1 1],c1);patch([0 1 1 1-e 1-e 0+e],[0 0 1 1-e 0+e 0+e],c2);patch([0 0 1 1-e 0+e 0+e],[0 1 1 1-e 1-e 0+e],c3);plot([0 1 1 0 0],[0 0 1 1 0]);disp('weights');
  "IW{3,2}(2,:)'" : Constant  Value=[0.445211164821717797490663315329584293067455291748046875;0.2497172286753712444618003019058960489928722381591796875;0.24675394014089579997062173788435757160186767578125;-0.017453169559885635397922243328139302320778369903564453125;-0.534125695750038431697248597629368305206298828125;0.041939997232147328831697308260118006728589534759521484375;0.475153394142820373335922568003297783434391021728515625]
      mask Display: e = 0.06;c1 = [120 150 230]/255;c2 = ([120 150 230]+0)/383;c3 = ([120 150 230]+128)/383;patch([0 1 1 0],[0 0 1 1],c1);patch([0 1 1 1-e 1-e 0+e],[0 0 1 1-e 0+e 0+e],c2);patch([0 0 1 1-e 0+e 0+e],[0 1 1 1-e 1-e 0+e],c3);plot([0 1 1 0 0],[0 0 1 1 0]);disp('weights');
  Mux : Mux  Inputs=2
      mask Display: e = 0.06;c1 = [120 150 230]/255;c2 = ([120 150 230]+0)/383;c3 = ([120 150 230]+128)/383;patch([0 1 1 0],[0 0 1 1],c1);patch([0 1 1 1-e 1-e 0+e],[0 0 1 1-e 0+e 0+e],c2);patch([0 0 1 1-e 0+e 0+e],[0 1 1 1-e 1-e 0+e],c3);plot([0 1 1 0 0],[0 0 1 1 0]);disp('Mux');
  dotprod1 : neural/Weight Functions/dotprod
  dotprod2 : neural/Weight Functions/dotprod
  "lz{3,2}" : Outport
      mask Display: e = 0.06;c1 = [120 230 180]/255;c2 = ([120 230 180]+0)/(256+128);c3 = ([120 230 180]+128)/(256+128);patch([0 1 1 0],[0 0 1 1],c1);patch([0 1 1 1-e 1-e 0+e],[0 0 1 1-e 0+e 0+e],c2);patch([0 0 1 1-e 0+e 0+e],[0 1 1 1-e 1-e 0+e],c3);plot([0 1 1 0 0],[0 0 1 1 0]);
  wires:
  Mux/1 -> "lz{3,2}"/1
  dotprod2/1 -> Mux/2
  "IW{3,2}(2,:)'"/1 -> dotprod2/1
  dotprod1/1 -> Mux/1
  "ad{3,2}"/1 -> dotprod2/2, dotprod1/2
  "IW{3,2}(1,:)'"/1 -> dotprod1/1

== matlab function ackerman_modelo_parte1_neuronal/ROS Robot/Conversion_diff_ackerman ==
  data: steering_wheel_angle input; V output; linear_vel_ackerman_kmh input; W output
function [V,W] = fcn(steering_wheel_angle, linear_vel_ackerman_kmh)

    %Aproximacion de angulo volante y velocidad linal a vel_linar y angular.
    % *************************************
    
    min_turning_radius_vehicle = 2;  % radio de giro del vehiculo. Radio minimo en el que gira 180 grados. 
    max_turning_radius_vehicle = 34; % radio de giro del vehiculo. Radio máximo con el volante girado 1º
    max_steering_wheel_angle = 90;  % angulo máximo de volante permitido (grados).
    max_vehicle_linear_speed = 30;  % velocidad máxima de vehiculo (km/h).
    
    
    % Filtrado des los valores máximos
    
    if steering_wheel_angle > max_steering_wheel_angle
        steering_wheel_angle = max_steering_wheel_angle;  
    end
    
    if steering_wheel_angle < (-1*max_steering_wheel_angle)
        steering_wheel_angle = max_steering_wheel_angle;  
    end
    
    if linear_vel_ackerman_kmh > max_vehicle_linear_speed
        linear_vel_ackerman_kmh = max_vehicle_linear_speed;
    end
    
    
    %Conversion a m/s
    linear_vel_ackerman_ms = linear_vel_ackerman_kmh/3.6; %(m/s)
    
    %Conversion a linear and angular velocity for the simulator.
    % v=rω --> ω = v/r
    
    % max_steering_wheel_angle -- > min_turning_radius_vehicle
    % steering_wheel_angle = 0 --> angular_vel_vehicle = 0;
    
    turning_radius = (max_turning_radius_vehicle-((max_turning_radius_vehicle-min_turning_radius_vehicle)/max_steering_wheel_angle)*abs(steering_wheel_angle));
    
    if steering_wheel_angle > 0
            turning_radius = turning_radius;
    elseif steering_wheel_angle < 0
            turning_radius = -1*turning_radius;
    end
    
    if abs(steering_wheel_angle) < 0.01
        angular_vel_vehicle = 0;
    else
        angular_vel_vehicle = linear_vel_ackerman_ms / turning_radius;
    end
    
    %Sin velocidad linear, tampoco debe girar
    
    if linear_vel_ackerman_ms == 0
        angular_vel_vehicle = 0;
    end
    
    
    %Rellenamos los campos del mensaje V y W
    V= linear_vel_ackerman_ms;

    W=angular_vel_vehicle;
    
    
    %********************************************************

== matlab function ackerman_modelo_parte1_neuronal/ROS Robot/MATLAB Function ==
  data: u input; y output
function y = fcn(u)
u(isinf(u))=5.0;
y = u;

== matlab function ackerman_modelo_parte1_neuronal/Condicion de Parada ==
  data: flag_parada output; raw_speed input; filter_speed output; sonar_2 input; sonar_3 input; sonar_8 input; sonar_9 input
function [flag_parada, filter_speed] = condicion_parada(raw_speed, sonar_2, sonar_3, sonar_8, sonar_9)

% Condicion de parada:
% - debeis decidir cuando se finaliza la maniobra de aparcamiento en base
%  a la información disponible:
%      - velocidad_lineal
%      - ángulo de volante      
%      - sensores
% Una vez que decidais cual es el criterio de parada debeis:
%   - Parar el vehículo con v_lineal = 0.
%   - Activar el flag_parada a 1 para indicar que ha finalizado la maniobra.

if sonar_2 >= 4 && sonar_3 >= 4 && sonar_8 < 1.3 && sonar_9 < 1.3 % Ejemplo de condición de parada

    %Es necesario parar el vehículo con v_lineal = 0 y activar el
    %flag_parada a 1 para indicar que ha finalizado la maniobra.
    filter_speed = 0.0;
    flag_parada=1;

else
    filter_speed = raw_speed;
    flag_parada=0;
end

== matlab function ackerman_modelo_parte1_neuronal/Evaluacion_maniobra/Evaluacion_fin_maniobra ==
  data: clock input; flag_parada input; x input; y input; theta input; stop_flag output
function stop_flag = evaluacion_maniobra(clock, flag_parada, x, y, theta)

if flag_parada == 1

    parking_time = clock
    parking_position_x = x
    parking_position_y = y
    parking_position_theta = theta
    stop_flag = 1;
else
    stop_flag = 0;

end
